simulink model "QPSK"  (R2023b)
settings: Solver=VariableStepAuto  StartTime=0.0  StopTime=50  RelTol=1e-3
libraries: commrflib2 x3, commrandsrc3 x1
settings Model: Creator=HP  LastModifiedBy=HP

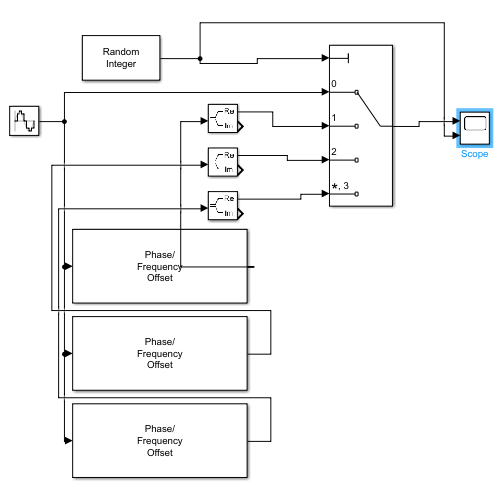
[thumbnail: Simulink's stored preview of the top-level diagram]
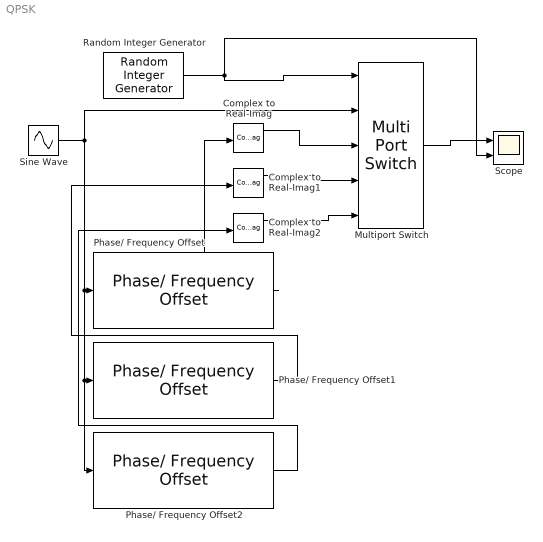
== system QPSK ==
  Complex to Real-Imag : ComplexToRealImag
  Complex to Real-Imag1 : ComplexToRealImag
  Complex to Real-Imag2 : ComplexToRealImag
  Multiport Switch : MultiPortSwitch  DataPortOrder=Zero-based contiguous  Inputs=4  DiagnosticForDefault=None  zeroidx=on  SaturateOnIntegerOverflow=off  InputSameDT=off
      settings: LockScale=on
  Phase/ Frequency Offset : commrflib2/Phase// Frequency Offset  phaseOffset=90  freqPort=off  freqOffset=0
      settings: LibrarySourceBlock=|
      | commrfcorlib/Phase//
      | Frequency
      | Offset
  Phase/ Frequency Offset1 : commrflib2/Phase// Frequency Offset  phaseOffset=180  freqPort=off  freqOffset=0
      settings: LibrarySourceBlock=|
      | commrfcorlib/Phase//
      | Frequency
      | Offset
  Phase/ Frequency Offset2 : commrflib2/Phase// Frequency Offset  phaseOffset=270  freqPort=off  freqOffset=0
      settings: LibrarySourceBlock=|
      | commrfcorlib/Phase//
      | Frequency
      | Offset
  Random Integer Generator : commrandsrc3/Random Integer Generator  SetSize=3  SeedSource=Auto  Seed=0  SampleTime=0.25  SamplesPerFrame=1  OutputDataType=uint8  SimulateUsing=Interpreted execution
  Scope : Scope  NumInputPorts=2
  Sine Wave : Sin  Frequency=2*pi  SampleTime=0.01
  wires:
  Sine Wave/1 -> Phase/ Frequency Offset2/1, Phase/ Frequency Offset1/1, Phase/ Frequency Offset/1, Multiport Switch/2
  Phase/ Frequency Offset/1 -> Complex to Real-Imag/1
  Phase/ Frequency Offset1/1 -> Complex to Real-Imag1/1
  Phase/ Frequency Offset2/1 -> Complex to Real-Imag2/1
  Complex to Real-Imag/1 -> Multiport Switch/3
  Complex to Real-Imag1/1 -> Multiport Switch/4
  Complex to Real-Imag2/1 -> Multiport Switch/5
  Random Integer Generator/1 -> Multiport Switch/1, Scope/2
  Multiport Switch/1 -> Scope/1
